simulink model "hil14_test"  (Simulink 7.0)
settings: Solver=ode45  StartTime=0.0  StopTime=100  MaxStep=0.01  RelTol=1e-3
PreLoadFcn:
  | eng_mdl_demo_v14_setup
InitFcn:
  | eng_mdl_demo_v14_setup
values from neighbouring files (symbols this model uses):
  amb =     [ws.mat]
  cylinder =     [ws.mat]
  fuel =     [ws.mat]
  im =     [ws.mat]
  MDL =     [ws.mat]
undefined symbols (not defined in the file or in its folder): notex
libraries: ni_annotations_lib x8, hil14_mdl_lib x3, simulink x1
CloseFcn:
  | eng_mdl_demo_v14_close
settings Model: Creator=Eric Bradley  LastModifiedBy=Eric Bradley  MotoHawkBuildVersion=000

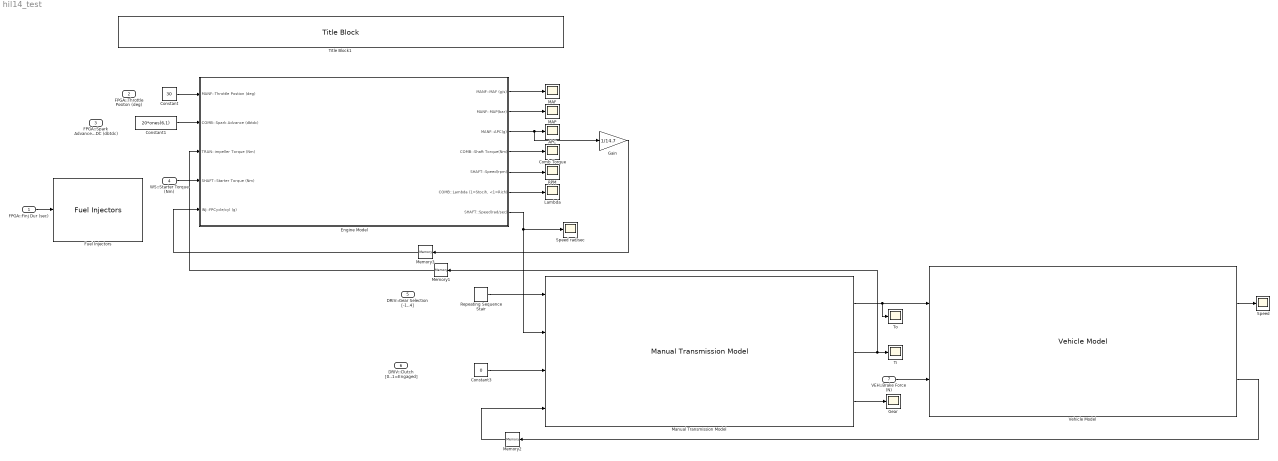
== system hil14_test ==
  FPGA::Finj Dur (sec) : Inport  OutDataType=sfix(16)  OutScaling=2^0
  FPGA::Throttle Positon (deg) : Inport  Port=2  OutDataType=sfix(16)  OutScaling=2^0
  FPGA::Spark Advance from Local TDC (dbtdc) : Inport  Port=3  OutDataType=sfix(16)  OutScaling=2^0
  WS::Starter Torque (Nm) : Inport  Port=4  OutDataType=sfix(16)  OutScaling=2^0
  DRIV::Gear Selection [-1..4] : Inport  Port=5  OutDataType=sfix(16)  OutScaling=2^0
  DRIV::Clutch [0..1=Engaged] : Inport  Port=6  OutDataType=sfix(16)  OutScaling=2^0
  VEH::Brake Force (N) : Inport  Port=7  OutDataType=sfix(16)  OutScaling=2^0
  APC : Scope
      settings: YMin=0  YMax=275  SaveName=ScopeData5
  Comb Torque : Scope
      settings: SaveName=ScopeData4
  Constant : Constant  Value=30  OutDataType=sfix(16)  OutScaling=2^0
  Constant1 : Constant  Value=20*ones(6,1)  OutDataType=sfix(16)  OutScaling=2^0
  Constant3 : Constant  Value=0  OutDataType=sfix(16)  OutScaling=2^0
  Engine Model : Subsystem  AncestorBlock=hil14_mdl_lib/Engine Model  mask{iname='engine.jpg'}
      mask prompts: iname "Image"
      mask init:
      | blk = gcb;
      | 
      | p = get_param(blk,'Position');
      | 
      | wd = p(3)-p(1);
      | ht = p(4)-p(2);
      | 
      | ar = wd/ht;
      | 
      | img = imread(iname);
      | ii = imfinfo(iname);
      | 
      | iar = ii.Width/ii.Height;
      | 
      | scale = 0.125;
      settings: OpenFcn=open_system(gcb,'Force')
      mask Display: image(img, [0.5-ii.Width/wd*scale/2, 0.5-ii.Height/ht*scale/2, ii.Width/wd*scale,ii.Height/ht*scale]);
  Fuel Injectors : hil14_mdl_lib/Fuel Injectors  SystemSampleTime=-1  iname='pfi.jpg'  scale=0.125
  Gain : Gain  Gain=1/14.7  ParameterDataType=sfix(16)  ParameterScaling=2^0  OutDataType=sfix(16)  OutScaling=2^0
  Gear : Scope
      settings: TimeRange=100  YMin=0  YMax=2  SaveName=ScopeData9
  Lambda : Scope
      settings: SaveName=ScopeData3
  MAF : Scope
  MAP : Scope
  Manual Transmission Model : hil14_mdl_lib/Manual Transmission Model  SystemSampleTime=-1  iname='Manual_Transmission.png'  scale=0.55
  Memory1 : Memory  Orientation=left  InheritSampleTime=on
  Memory2 : Memory  Orientation=left  InheritSampleTime=on
  Memory3 : Memory  Orientation=left  InheritSampleTime=on
  RPM : Scope
      settings: YMin=0  YMax=6500  SaveName=ScopeData2
  Repeating Sequence Stair : simulink/Sources/Repeating Sequence Stair  SystemSampleTime=-1  OutValues=[1 2 3 4 4 4 3 2 1]  tsamp=4  OutMin=[]  OutMax=[]  OutDataTypeStr=float('double')  OutputDataTypeScalingMode=Specify via dialog  OutDataType=float('double')  ConRadixGroup=Best Precision: Vector-wise  OutScaling=2^-12
  Speed : Scope
      settings: TimeRange=100  YMin=0  YMax=35  SaveName=ScopeData6
  Speed rad/sec : Scope
      settings: SaveName=ScopeData10
  Ti : Scope
      settings: YMin=0  YMax=6500  SaveName=ScopeData7
  Title Block1 : ni_annotations_lib/Title Block  SystemSampleTime=-1  tx_title=notex(get_param(gcs,'Name'))
  To : Scope
      settings: YMin=0  YMax=6500  SaveName=ScopeData8
  Vehicle Model : hil14_mdl_lib/Vehicle Model  SystemSampleTime=-1  iname='veh.jpg'  scale=0.5
  wires:
  WS::Starter Torque (Nm)/1 -> Engine Model/4(SHAFT::Starter Torque (Nm))
  Engine Model/3(MANF::APC(g)) -> APC/1, Gain/1
  Engine Model/1(MANF::MAF (g/s)) -> MAF/1
  Engine Model/2(MANF::MAP(bar)) -> MAP/1
  Engine Model/5(SHAFT::Speed(rpm)) -> RPM/1
  Engine Model/6("COMB::Lambda (1=Stocih, <1=Rich)") -> Lambda/1
  Engine Model/4(COMB::Shaft Torque(Nm)) -> Comb Torque/1
  Engine Model/7(SHAFT::Speed(rad/sec)) -> Manual Transmission Model/2, Speed rad/sec/1
  Manual Transmission Model/2 -> Ti/1, Memory1/1
  Manual Transmission Model/1 -> To/1, Vehicle Model/1
  Manual Transmission Model/3 -> Gear/1
  VEH::Brake Force (N)/1 -> Vehicle Model/2
  Vehicle Model/2 -> Memory2/1
  Memory1/1 -> Engine Model/3(TRAN::impeller Torque (Nm))
  Memory2/1 -> Manual Transmission Model/4
  FPGA::Finj Dur (sec)/1 -> Fuel Injectors/1
  Vehicle Model/1 -> Speed/1
  Repeating Sequence Stair/1 -> Manual Transmission Model/1
  Constant3/1 -> Manual Transmission Model/3
  Gain/1 -> Memory3/1
  Constant/1 -> Engine Model/1(MANF::Throttle Postion (deg))
  Constant1/1 -> Engine Model/2(COMB::Spark Advance (dbtdc))
  Memory3/1 -> Engine Model/5(INJ::FPCycle/cyl (g))

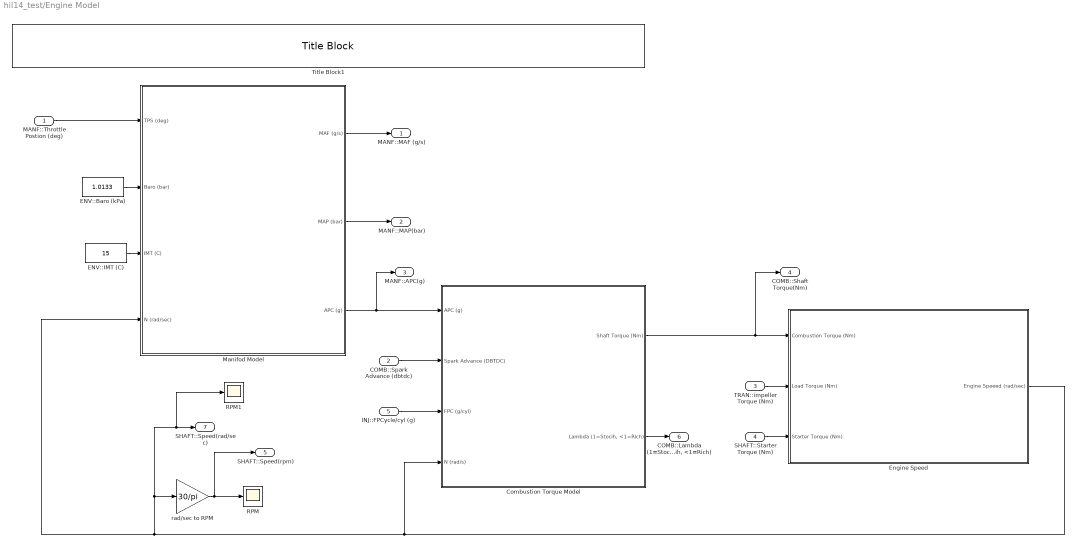
== system hil14_test/Engine Model ==
  MANF::Throttle Postion (deg) : Inport  OutDataType=sfix(16)  OutScaling=2^0
  COMB::Spark Advance (dbtdc) : Inport  Port=2  PortDimensions=6  OutDataType=sfix(16)  OutScaling=2^0
  TRAN::impeller Torque (Nm) : Inport  Port=3  OutDataType=sfix(16)  OutScaling=2^0
  SHAFT::Starter Torque (Nm) : Inport  Port=4  OutDataType=sfix(16)  OutScaling=2^0
  INJ::FPCycle/cyl (g) : Inport  Port=5  OutDataType=sfix(16)  OutScaling=2^0
  Combustion Torque Model : Subsystem  mask{iname='cylinder.jpg'}
      mask prompts: iname "Image"
      mask init:
      | blk = gcb;
      | 
      | p = get_param(blk,'Position');
      | 
      | wd = p(3)-p(1);
      | ht = p(4)-p(2);
      | 
      | ar = wd/ht;
      | 
      | img = imread(iname);
      | ii = imfinfo(iname);
      | 
      | iar = ii.Width/ii.Height;
      settings: OpenFcn=open_system(gcb,'Force')
      mask Display: image(img, [0.5-ii.Width/wd*0.125/2, 0.5-ii.Height/ht*0.125/2, ii.Width/wd*0.125,ii.Height/ht*0.125]);
  ENV::Baro (kPa) : Constant  Value=1.0133  OutDataType=sfix(16)  OutScaling=2^0
  ENV::IMT (C) : Constant  Value=15  OutDataType=sfix(16)  OutScaling=2^0
  Engine Speed : Subsystem  mask{iname='piston.jpg'}
      mask prompts: iname "Image"
      mask init:
      | blk = gcb;
      | 
      | p = get_param(blk,'Position');
      | 
      | wd = p(3)-p(1);
      | ht = p(4)-p(2);
      | 
      | ar = wd/ht;
      | 
      | img = imread(iname);
      | ii = imfinfo(iname);
      | 
      | iar = ii.Width/ii.Height;
      settings: OpenFcn=open_system(gcb,'Force')
      mask Display: image(img, [0.5-ii.Width/wd*0.5/2, 0.5-ii.Height/ht*0.5/2, ii.Width/wd*0.5,ii.Height/ht*0.5]);
  Manifod Model : Subsystem  mask{iname='intake_manifold.jpg'}
      mask prompts: iname "Image"
      mask init:
      | blk = gcb;
      | 
      | p = get_param(blk,'Position');
      | 
      | wd = p(3)-p(1);
      | ht = p(4)-p(2);
      | 
      | ar = wd/ht;
      | 
      | img = imread(iname);
      | ii = imfinfo(iname);
      | 
      | iar = ii.Width/ii.Height;
      settings: OpenFcn=open_system(gcb,'Force')
      mask Display: image(img, [0.5-ii.Width/wd*0.25/2, 0.5-ii.Height/ht*0.25/2, ii.Width/wd*0.25,ii.Height/ht*0.25]);
  RPM : Scope
      settings: YMin=1100  YMax=2200  SaveName=ScopeData8
  RPM1 : Scope
      settings: YMin=1100  YMax=2200  SaveName=ScopeData14
  Title Block1 : ni_annotations_lib/Title Block  SystemSampleTime=-1  tx_title=get_param(gcs,'Name')
  rad/sec to RPM : Gain  Gain=30/pi  ParameterDataType=sfix(16)  ParameterScaling=2^0  OutDataType=sfix(16)  OutScaling=2^0
  MANF::MAF (g/s) : Outport  OutDataType=sfix(16)  OutScaling=2^0
  MANF::MAP(bar) : Outport  Port=2  OutDataType=sfix(16)  OutScaling=2^0
  MANF::APC(g) : Outport  Port=3  OutDataType=sfix(16)  OutScaling=2^0
  COMB::Shaft Torque(Nm) : Outport  Port=4  OutDataType=sfix(16)  OutScaling=2^0
  SHAFT::Speed(rpm) : Outport  Port=5  OutDataType=sfix(16)  OutScaling=2^0
  "COMB::Lambda (1=Stocih, <1=Rich)" : Outport  Port=6  OutDataType=sfix(16)  OutScaling=2^0
  SHAFT::Speed(rad/sec) : Outport  Port=7  OutDataType=sfix(16)  OutScaling=2^0
  wires:
  ENV::Baro (kPa)/1 -> Manifod Model/2(Baro (bar))
  ENV::IMT (C)/1 -> Manifod Model/3(IMT (C))
  Manifod Model/1(MAF (g/s)) -> MANF::MAF (g/s)/1
  Manifod Model/2(MAP (bar)) -> MANF::MAP(bar)/1
  Manifod Model/3(APC (g)) -> MANF::APC(g)/1, Combustion Torque Model/1(APC (g))
  Combustion Torque Model/1(Shaft Torque (Nm)) -> Engine Speed/1(Combustion Torque (Nm)), COMB::Shaft Torque(Nm)/1
  rad/sec to RPM/1 -> RPM/1, SHAFT::Speed(rpm)/1
  Engine Speed/1(Engine Speeed (rad/sec)) -> Manifod Model/4(N (rad/sec)), rad/sec to RPM/1, SHAFT::Speed(rad/sec)/1, RPM1/1, Combustion Torque Model/4(N (rad/s))
  MANF::Throttle Postion (deg)/1 -> Manifod Model/1(TPS (deg))
  Combustion Torque Model/2("Lambda (1=Stocih, <1=Rich)") -> "COMB::Lambda (1=Stocih, <1=Rich)"/1
  COMB::Spark Advance (dbtdc)/1 -> Combustion Torque Model/2(Spark Advance (DBTDC))
  TRAN::impeller Torque (Nm)/1 -> Engine Speed/2(Load Torque (Nm))
  SHAFT::Starter Torque (Nm)/1 -> Engine Speed/3(Starter Torque (Nm))
  INJ::FPCycle/cyl (g)/1 -> Combustion Torque Model/3(FPC (g/cyl))

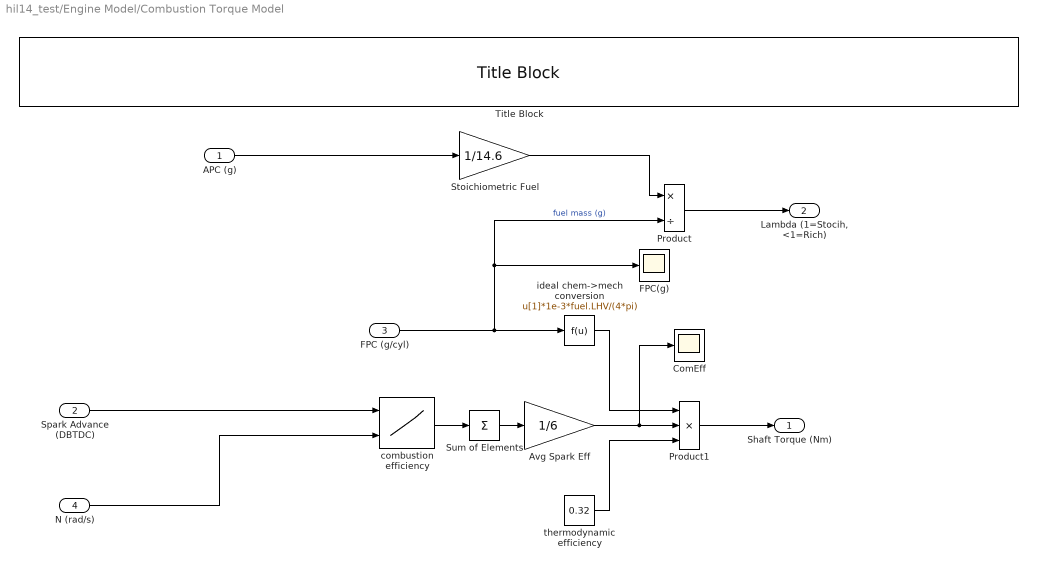
== system hil14_test/Engine Model/Combustion Torque Model ==
  APC (g) : Inport  OutDataType=sfix(16)  OutScaling=2^0
  Spark Advance (DBTDC) : Inport  Port=2  OutDataType=sfix(16)  OutScaling=2^0
  FPC (g/cyl) : Inport  Port=3  OutDataType=sfix(16)  OutScaling=2^0
  N (rad/s) : Inport  Port=4  PortDimensions=1  OutDataType=sfix(16)  OutScaling=2^0
  Avg Spark Eff : Gain  Gain=1/6  ParameterDataType=sfix(16)  ParameterScaling=2^0  OutDataType=sfix(16)  OutScaling=2^0  SaturateOnIntegerOverflow=on
  ComEff : Scope
      settings: SaveName=ScopeData10
  FPC(g) : Scope
      settings: SaveName=ScopeData7
  Product : Product  Inputs=*/  OutDataType=sfix(16)  OutScaling=2^0  SaturateOnIntegerOverflow=on
  Product1 : Product  Inputs=3  OutDataType=sfix(16)  OutScaling=2^0  SaturateOnIntegerOverflow=on
  Stoichiometric Fuel : Gain  Gain=1/14.6  ParameterDataType=sfix(16)  ParameterScaling=2^0  OutDataType=sfix(16)  OutScaling=2^0  SaturateOnIntegerOverflow=on
  Sum of Elements : Sum  Inputs=+  OutDataType=sfix(16)  OutScaling=2^-10
  Title Block : ni_annotations_lib/Title Block  SystemSampleTime=-1  tx_title=get_param(gcs,'Name')
  combustion efficiency : Lookup2D  RowIndex=cylinder.ce.spark_timing  ColumnIndex=cylinder.ce.rpm*pi/30  Table=cylinder.ce.table  LookUpMeth=Interpolation-Use End Values  OutDataType=sfix(16)  OutScaling=2^0  SaturateOnIntegerOverflow=on
  ideal chem->mech conversion : Fcn  Expr=u[1]*1e-3*fuel.LHV/(4*pi)
  thermodynamic efficiency : Constant  Value=0.32  OutDataType=sfix(16)  OutScaling=2^0
  Shaft Torque (Nm) : Outport  OutDataType=sfix(16)  OutScaling=2^0
  "Lambda (1=Stocih, <1=Rich)" : Outport  Port=2  OutDataType=sfix(16)  OutScaling=2^0
  wires:
  N (rad/s)/1 -> combustion efficiency/2
  Spark Advance (DBTDC)/1 -> combustion efficiency/1
  FPC (g/cyl)/1 -> ideal chem->mech conversion/1, FPC(g)/1, Product/2  "fuel mass (g)"
  combustion efficiency/1 -> Sum of Elements/1
  ideal chem->mech conversion/1 -> Product1/1
  thermodynamic efficiency/1 -> Product1/3
  Product1/1 -> Shaft Torque (Nm)/1
  APC (g)/1 -> Stoichiometric Fuel/1
  Stoichiometric Fuel/1 -> Product/1
  Product/1 -> "Lambda (1=Stocih, <1=Rich)"/1
  Sum of Elements/1 -> Avg Spark Eff/1
  Avg Spark Eff/1 -> Product1/2, ComEff/1

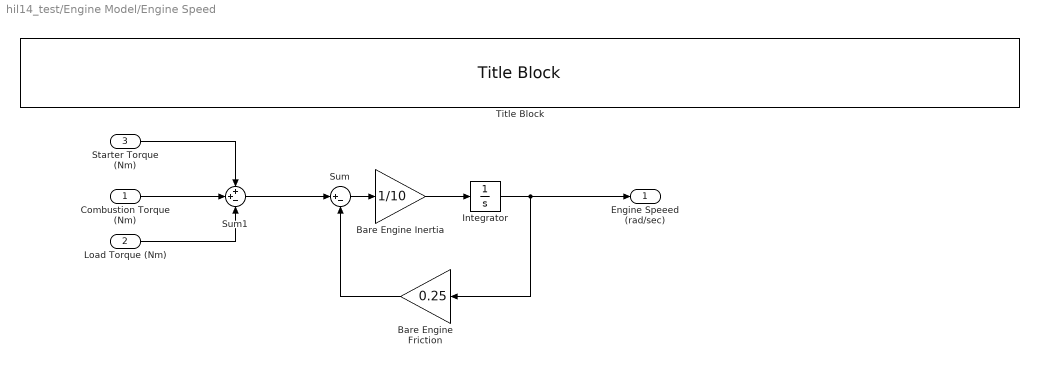
== system hil14_test/Engine Model/Engine Speed ==
  Combustion Torque (Nm) : Inport  OutDataType=sfix(16)  OutScaling=2^0
  Load Torque (Nm) : Inport  Port=2  OutDataType=sfix(16)  OutScaling=2^0
  Starter Torque (Nm) : Inport  Port=3  OutDataType=sfix(16)  OutScaling=2^0
  Bare Engine Friction : Gain  Orientation=left  Gain=0.25  ParameterDataType=sfix(16)  ParameterScaling=2^0  OutDataType=sfix(16)  OutScaling=2^0
  Bare Engine Inertia : Gain  Gain=1/10  ParameterDataType=sfix(16)  ParameterScaling=2^0  OutDataType=sfix(16)  OutScaling=2^0
  Integrator : Integrator  InitialCondition=600*pi/30  LimitOutput=on  UpperSaturationLimit=1000  LowerSaturationLimit=0
  Sum : Sum  Inputs=|+-  OutDataType=sfix(16)  OutScaling=2^0
  Sum1 : Sum  Inputs=++-  OutDataType=sfix(16)  OutScaling=2^0
  Title Block : ni_annotations_lib/Title Block  SystemSampleTime=-1  tx_title=get_param(gcs,'Name')
  Engine Speeed (rad/sec) : Outport  OutDataType=sfix(16)  OutScaling=2^0
  wires:
  Sum/1 -> Bare Engine Inertia/1
  Bare Engine Inertia/1 -> Integrator/1
  Integrator/1 -> Engine Speeed (rad/sec)/1, Bare Engine Friction/1
  Bare Engine Friction/1 -> Sum/2
  Load Torque (Nm)/1 -> Sum1/3
  Combustion Torque (Nm)/1 -> Sum1/2
  Sum1/1 -> Sum/1
  Starter Torque (Nm)/1 -> Sum1/1

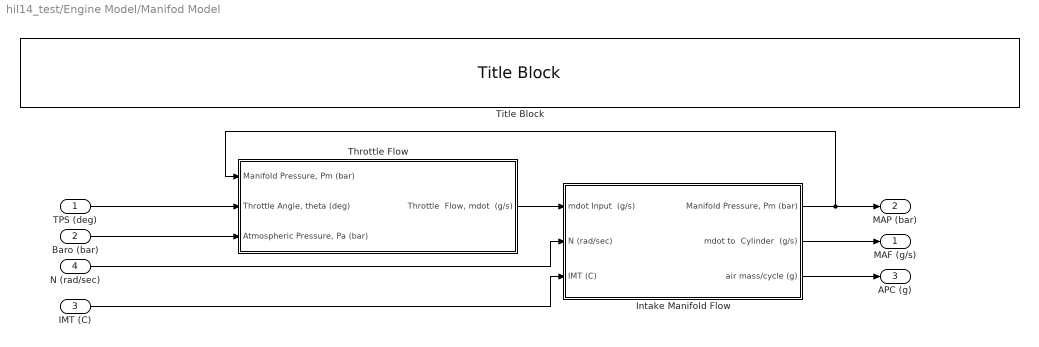
== system hil14_test/Engine Model/Manifod Model ==
  TPS (deg) : Inport  OutDataType=sfix(16)  OutScaling=2^0
  Baro (bar) : Inport  Port=2  OutDataType=sfix(16)  OutScaling=2^0
  IMT (C) : Inport  Port=3  OutDataType=sfix(16)  OutScaling=2^0
  N (rad/sec) : Inport  Port=4  OutDataType=sfix(16)  OutScaling=2^0
  Intake Manifold Flow : Subsystem
  Throttle Flow : Subsystem
  Title Block : ni_annotations_lib/Title Block  SystemSampleTime=-1  tx_title=get_param(gcs,'Name')
  MAF (g/s) : Outport  OutDataType=sfix(16)  OutScaling=2^0
  MAP (bar) : Outport  Port=2  OutDataType=sfix(16)  OutScaling=2^0
  APC (g) : Outport  Port=3  OutDataType=sfix(16)  OutScaling=2^0
  wires:
  TPS (deg)/1 -> Throttle Flow/2("Throttle Angle, theta (deg)")
  IMT (C)/1 -> Intake Manifold Flow/3(IMT (C))
  N (rad/sec)/1 -> Intake Manifold Flow/2(N (rad/sec))
  Baro (bar)/1 -> Throttle Flow/3("Atmospheric Pressure, Pa (bar) ")
  Throttle Flow/1("Throttle  Flow, mdot  (g/s)") -> Intake Manifold Flow/1(mdot Input  (g/s))
  Intake Manifold Flow/2(mdot to  Cylinder  (g/s)) -> MAF (g/s)/1
  Intake Manifold Flow/3(air mass/cycle (g)) -> APC (g)/1
  Intake Manifold Flow/1("Manifold Pressure, Pm (bar)") -> MAP (bar)/1, Throttle Flow/1("Manifold Pressure, Pm (bar)")

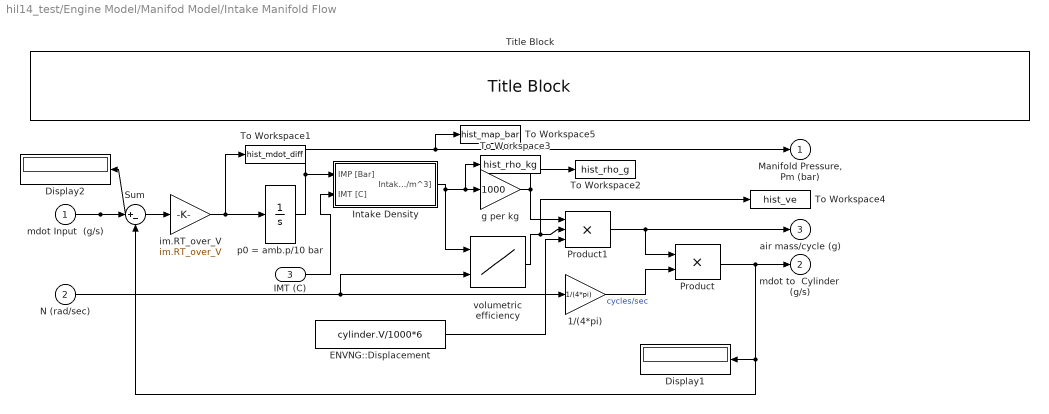
== system hil14_test/Engine Model/Manifod Model/Intake Manifold Flow ==
  mdot Input  (g/s) : Inport  OutDataType=sfix(16)  OutScaling=2^0
  N (rad/sec) : Inport  Port=2  OutDataType=sfix(16)  OutScaling=2^0
  IMT (C) : Inport  Port=3  OutDataType=sfix(16)  OutScaling=2^0
  1/(4*pi) : Gain  Gain=1/(4*pi)  ParameterDataType=sfix(16)  ParameterScaling=2^0  OutDataType=sfix(16)  OutScaling=2^0  SaturateOnIntegerOverflow=on
  Display1 : Display
  Display2 : Display
  ENVNG::Displacement : Constant  Value=cylinder.V/1000*6  OutDataType=sfix(16)  OutScaling=2^0
  Intake Density : Subsystem
  Product : Product  OutDataType=sfix(16)  OutScaling=2^0  SaturateOnIntegerOverflow=on
  Product1 : Product  Inputs=3  OutDataType=sfix(16)  OutScaling=2^0  SaturateOnIntegerOverflow=on
  Sum : Sum  Inputs=|+-  OutDataType=sfix(16)  OutScaling=2^0  SaturateOnIntegerOverflow=on  InputSameDT=on
  Title Block : ni_annotations_lib/Title Block  SystemSampleTime=-1  tx_title=get_param(gcs,'Name')
  To Workspace1 : ToWorkspace  VariableName=hist_mdot_diff  SampleTime=-1  SaveFormat=Array
      settings: MaxDataPoints=hist_sample_size
  To Workspace2 : ToWorkspace  VariableName=hist_rho_g  SampleTime=-1  SaveFormat=Array
      settings: MaxDataPoints=hist_sample_size
  To Workspace3 : ToWorkspace  VariableName=hist_rho_kg  SampleTime=-1  SaveFormat=Array
      settings: MaxDataPoints=hist_sample_size
  To Workspace4 : ToWorkspace  VariableName=hist_ve  SampleTime=-1  SaveFormat=Array
      settings: MaxDataPoints=hist_sample_size
  To Workspace5 : ToWorkspace  VariableName=hist_map_bar  SampleTime=-1  SaveFormat=Array
      settings: MaxDataPoints=hist_sample_size
  g per kg : Gain  Gain=1000  ParameterDataType=sfix(16)  ParameterScaling=2^0  OutDataType=sfix(16)  OutScaling=2^0  SaturateOnIntegerOverflow=on
  im.RT_over_V : Gain  Gain=im.RT_over_V  ParameterDataType=sfix(16)  ParameterScaling=2^0  OutDataType=sfix(16)  OutScaling=2^0  SaturateOnIntegerOverflow=on
  p0 = amb.p/10 bar : Integrator  InitialCondition=amb.p*0.99  LimitOutput=on  UpperSaturationLimit=0.99*amb.p  LowerSaturationLimit=0.001*amb.p
  volumetric efficiency : Lookup2D  RowIndex=MDL.ENGINE.VolumetricEff.x  ColumnIndex=MDL.ENGINE.VolumetricEff.y  Table=0.7*MDL.ENGINE.VolumetricEff.v  LookUpMeth=Interpolation-Use End Values  OutDataType=sfix(16)  OutScaling=2^0  SaturateOnIntegerOverflow=on
  "Manifold Pressure, Pm (bar)" : Outport  InitialOutput=0
  mdot to  Cylinder  (g/s) : Outport  Port=2  InitialOutput=0
  air mass/cycle (g) : Outport  Port=3  InitialOutput=0
  wires:
  p0 = amb.p/10 bar/1 -> Intake Density/1(IMP [Bar]), "Manifold Pressure, Pm (bar)"/1, To Workspace5/1
  Sum/1 -> im.RT_over_V/1
  N (rad/sec)/1 -> volumetric efficiency/2, 1/(4*pi)/1
  im.RT_over_V/1 -> To Workspace1/1, p0 = amb.p/10 bar/1
  mdot Input  (g/s)/1 -> Sum/1, Display2/1
  volumetric efficiency/1 -> To Workspace4/1, Product1/2
  1/(4*pi)/1 -> Product/2  "cycles/sec"
  Product/1 -> mdot to  Cylinder  (g/s)/1, Sum/2, Display1/1
  Intake Density/1(Intake Density [Kg/m^3]) -> volumetric efficiency/1, g per kg/1, To Workspace3/1
  IMT (C)/1 -> Intake Density/2(IMT [C])
  Product1/1 -> air mass/cycle (g)/1, Product/1
  g per kg/1 -> Product1/1, To Workspace2/1
  ENVNG::Displacement/1 -> Product1/3

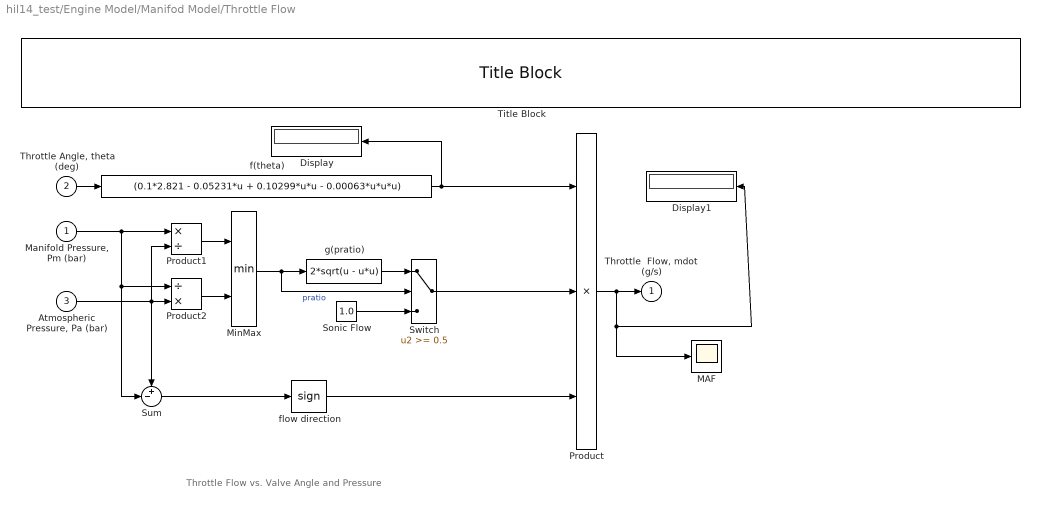
== system hil14_test/Engine Model/Manifod Model/Throttle Flow ==
  note: Throttle Flow vs. Valve Angle and Pressure
  "Manifold Pressure, Pm (bar)" : Inport  OutDataType=sfix(16)  OutScaling=2^0
  "Throttle Angle, theta (deg)" : Inport  Port=2  OutDataType=sfix(16)  OutScaling=2^0
  "Atmospheric Pressure, Pa (bar) " : Inport  Port=3  OutDataType=sfix(16)  OutScaling=2^0
  Display : Display
  Display1 : Display
  MAF : Scope
      settings: YMin=1.5  YMax=8.5  SaveName=ScopeData11
  MinMax : MinMax  Inputs=2  SaturateOnIntegerOverflow=on  InputSameDT=on
  Product : Product  Inputs=3  OutDataType=sfix(16)  OutScaling=2^0  SaturateOnIntegerOverflow=on  InputSameDT=on
  Product1 : Product  Inputs=*/  OutDataType=sfix(16)  OutScaling=2^0  SaturateOnIntegerOverflow=on  InputSameDT=on
  Product2 : Product  Inputs=/*  OutDataType=sfix(16)  OutScaling=2^0  SaturateOnIntegerOverflow=on  InputSameDT=on
  "Sonic Flow " : Constant  Value=1.0  OutDataType=sfix(16)  OutScaling=2^0
  Sum : Sum  Inputs=+-|  OutDataType=sfix(16)  OutScaling=2^0  SaturateOnIntegerOverflow=on  InputSameDT=on
  Switch : Switch  Threshold=0.5  SaturateOnIntegerOverflow=on  InputSameDT=on
  Title Block : ni_annotations_lib/Title Block  SystemSampleTime=-1  tx_title=get_param(gcs,'Name')
  f(theta) : Fcn  Expr=(0.1*2.821 - 0.05231*u + 0.10299*u*u - 0.00063*u*u*u)
  flow direction : Signum
  g(pratio) : Fcn  Expr=2*sqrt(u - u*u)
  "Throttle  Flow, mdot  (g/s)" : Outport  InitialOutput=0
  wires:
  f(theta)/1 -> Product/1, Display/1
  Product/1 -> "Throttle  Flow, mdot  (g/s)"/1, MAF/1, Display1/1
  "Throttle Angle, theta (deg)"/1 -> f(theta)/1
  MinMax/1 -> g(pratio)/1, Switch/2  "pratio"
  Sum/1 -> flow direction/1
  flow direction/1 -> Product/3
  Switch/1 -> Product/2
  "Sonic Flow "/1 -> Switch/3
  g(pratio)/1 -> Switch/1
  "Atmospheric Pressure, Pa (bar) "/1 -> Product1/2, Product2/2, Sum/1
  Product1/1 -> MinMax/1
  Product2/1 -> MinMax/2
  "Manifold Pressure, Pm (bar)"/1 -> Product1/1, Product2/1, Sum/2

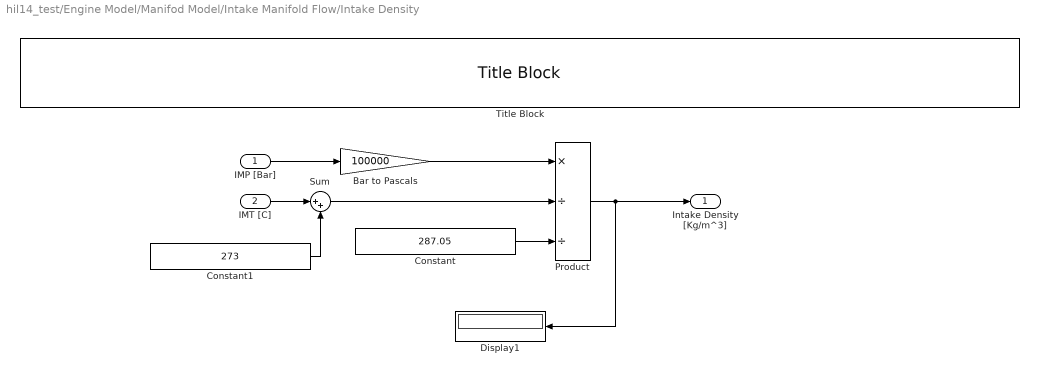
== system hil14_test/Engine Model/Manifod Model/Intake Manifold Flow/Intake Density ==
  IMP [Bar] : Inport  OutDataType=sfix(16)  OutScaling=2^0
  IMT [C] : Inport  Port=2  OutDataType=sfix(16)  OutScaling=2^0
  Bar to Pascals : Gain  Gain=100000  ParameterDataType=sfix(16)  ParameterScaling=2^0  OutDataType=sfix(16)  OutScaling=2^0
  Constant : Constant  Value=287.05  OutDataType=sfix(16)  OutScaling=2^0
  Constant1 : Constant  Value=273  OutDataType=sfix(16)  OutScaling=2^0
  Display1 : Display
  Product : Product  Inputs=*//  OutDataType=sfix(16)  OutScaling=2^0  RndMeth=Zero
  Sum : Sum  Inputs=|++  OutDataType=sfix(16)  OutScaling=2^0
  Title Block : ni_annotations_lib/Title Block  SystemSampleTime=-1  tx_title=get_param(gcs,'Name')
  Intake Density [Kg/m^3] : Outport  OutDataType=sfix(16)  OutScaling=2^0
  wires:
  Product/1 -> Intake Density [Kg/m^3]/1, Display1/1
  IMP [Bar]/1 -> Bar to Pascals/1
  Sum/1 -> Product/2
  Constant1/1 -> Sum/2
  IMT [C]/1 -> Sum/1
  Constant/1 -> Product/3
  Bar to Pascals/1 -> Product/1
